simulink model "task_2"  (R2024a)
settings: Solver=VariableStepAuto  StartTime=0.0  StopTime=30  RelTol=1e-3
settings Model: Creator=alexe  LastModifiedBy=alexe

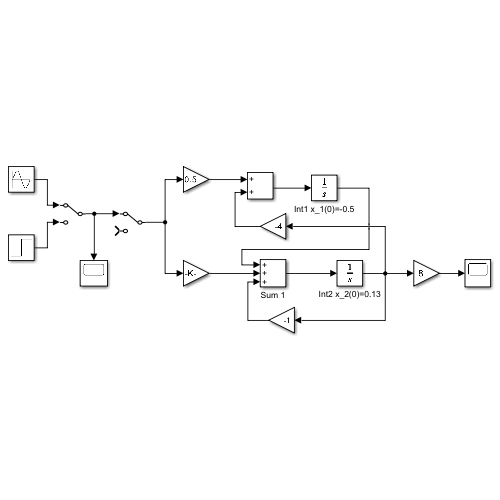
[thumbnail: Simulink's stored preview of the top-level diagram]
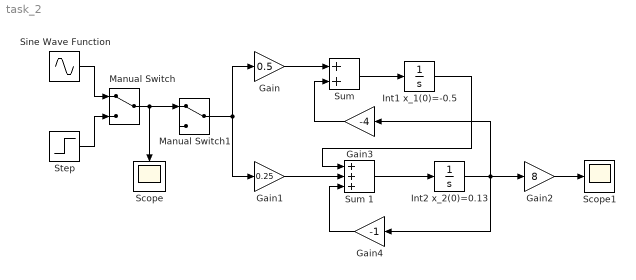
== system task_2 ==
  Gain : Gain  Gain=0.5
  Gain1 : Gain  Gain=0.25
  Gain2 : Gain  Gain=8
  Gain3 : Gain  Gain=-4
  Gain4 : Gain  Gain=-1
  Int1 x_1(0)=-0.5 : Integrator
  Int2 x_2(0)=0.13 : Integrator
  Manual Switch : ManualSwitch
  Manual Switch1 : ManualSwitch
  Scope : Scope
  Scope1 : Scope
  Sine Wave Function : Sin  Amplitude=2  SampleTime=0
  Step : Step  SampleTime=0
  Sum : Sum
  Sum 1 : Sum  Inputs=+++
  wires:
  Sine Wave Function/1 -> Manual Switch/1
  Step/1 -> Manual Switch/2
  Manual Switch/1 -> Scope/1, Manual Switch1/1
  Manual Switch1/1 -> Gain/1, Gain1/1
  Gain1/1 -> Sum 1/2
  Sum 1/1 -> Int2 x_2(0)=0.13/1
  Int2 x_2(0)=0.13/1 -> Gain4/1, Gain3/1, Gain2/1
  Gain/1 -> Sum/1
  Sum/1 -> Int1 x_1(0)=-0.5/1
  Gain3/1 -> Sum/2
  Int1 x_1(0)=-0.5/1 -> Sum 1/1
  Gain4/1 -> Sum 1/3
  Gain2/1 -> Scope1/1
